simulink model "TRIAD"  (R2017a)
settings: Solver=ode4  StartTime=0.0  StopTime=20000  FixedStep=0.1  RelTol=1e-3  EnableMultiTasking=on
undefined symbols (not defined in the file): mbaseserialmask, RxBuffer
libraries: xpcseriallib x17, vrlib x7, slrtlib x4, sharedtransform x3, sharedutil x2, dspinverses x2, dspmathops x2, simulink x1, dspsigops x1
(part 3 of 3)

== matlab function TRIAD/TRIAD_inner_use_Projection/BODY_TRIAD ==
  data: v input; c_triad output; w input
function c_triad = fcn(v, w)
    nz = norm(v);
    if (nz == 0)
        c_triad = eye(3);
    else
        x = v/norm(v);
        z = cross(x, w);
        z = z/norm(z);
        y = cross(z, x);
        c_triad = [x'; y'; z'];
    end
end

== matlab function TRIAD/SUN_function/Subsystem8/MATLAB Function4 ==
  data: djm input; sunpos output; ts input
function sunpos  = sun (djm, ts)
% [sunpos] = sun (djm, ts)
%
%	The subroutine sun calculates the position vector
%	of the Sun in the geocentric inertial system refered
%	to j2000 equator and equinox.
%
% Input:
%	djm
%		modified julian date in days, referred to 1950.0.
%	ts
%		fraction of the day in seconds.
%
% Output:
%	sunpos
%		position vector of the sun:
%		(1) - first component of earth-sun position vector in meters.
%		(2) - second component of earth-sun position vector in meters.
%		(3) - third component of earth-sun position vector in meters.
%		(4) - right ascension in radians.
%		(5) - declination in radians.
%		(6) - radius vector (distance) in meters.
%
% Remarks:
%	this subroutine is optimized from 1950-1-1 00:01:06
%	until year 2050.
%
% Author:
%	Helio Koiti Kuga and Ulisses T. V. Guedes * version 1.0
%	C version by Valdemir Carrara 7/05
%   Valdemir Carrara            March/09        Matlab

rad = pi/180;
ASTRONOMICAL_UNIT	= 149.60e+09;		% Astronomical unit (meters)

t = djm - 18262.5 + ts/86400.;%86400:1day second 
                              %18262.5 : J2000년도 Jan1 day1  
%	Long. media do sol, corrigida

alom_ab = mod ((280.460 + 0.9856474*t)*rad, 2*pi);
% 280.460 = mean longitude of the sun
% alom_ab : meanlongitude
% Sun's mean anomaly
% site : https://forum.logicmachine.net/showthread.php?tid=510

% alom_ab = 280.461 + 0.9856474 * t;
% while (alom_ab<0)
%     alom_ab = alom_ab + 360.0;
% end

if alom_ab < 0
    alom_ab = alom_ab + 2*pi;
end
% http://webcache.googleusercontent.com/search?q=cache:http://www.astro.uni.torun.pl/~kb/AllSky-old/Docs/Top2B2.htm&gws_rd=cr&dcr=0&ei=MUuaWu_oHYyB8gXs_J-4Ag
%	Anomalia media
% https://en.wikipedia.org/wiki/Position_of_the_Sun
an_mean = mod ((357.528 + 0.9856003*t)*rad, 2*pi);
if an_mean < 0
    an_mean = an_mean + 2*pi;
end

an_mean_2 = an_mean +  an_mean;

if an_mean_2 > 2*pi
    an_mean_2 = mod (an_mean_2, 2*pi);
end

ecli_lo = alom_ab + (1.915*sin(an_mean) +0.02*sin(an_mean_2))*rad;
sin_ecli_lo = sin(ecli_lo);
cos_ecli_lo = cos(ecli_lo);

%	ecliptic latitude	ecli_la = 0

obl_ecli = (23.439 - 4.e-7*t)*rad; % tilt angle 23.439
sin_obl_ecli = sin(obl_ecli);
cos_obl_ecli = cos(obl_ecli);

sunpos = [0, 0, 0, 0, 0, 0];
sunpos(4)  = atan2(cos_obl_ecli*sin_ecli_lo, cos_ecli_lo);
if sunpos(4) < 0
    sunpos(4) = sunpos(4) + 2*pi;
end

sunpos(5) = asin(sin_obl_ecli*sin_ecli_lo);
sunpos(6) = (1.00014 - 0.01671*cos(an_mean) - 1.4e-4*cos(an_mean_2))*ASTRONOMICAL_UNIT;

sunpos(1) = sunpos(6) * cos_ecli_lo;
sunpos(2) = sunpos(6) * cos_obl_ecli * sin_ecli_lo;
sunpos(3) = sunpos(6) * sin_obl_ecli * sin_ecli_lo;
end

== matlab function TRIAD/SUN_function/Subsystem8/MATLAB Function5 ==
  data: u input; y output
function y = fcn(u)
y = u(1:3);

end

== matlab function TRIAD/SUN_function/Subsystem8/MATLAB Function2 ==
  data: sat_pos input; shadow output; sun_pos input
function shadow  = earth_shadow (sat_pos, sun_pos)
% [shadow] = earth_shadow (sat_pos, sun_pos)
%
%	The function earth_shadow verifies if a given position
%	is or isn't in the earth shadow.
%
% Inputs:
%	sat_pos
%		spacecraft coordinates in the inertial system, in meters.
%	sun_pos
%		coordinates of the sun in the inertial frame, in meters.
%
% Remarks:
%	1 - Earth is considered as a sphere
%	2 - Penunbra is calculated as straight horizon line
%
% Outputs:
%	earth_shadow
%		0: spacecraft is in the earth shadow
%		1: spacecraft is illuminated by the sun
%       between 0 and 1: spacecraft is in the Earth penumbra,
%		earth_shadow gives the visible fraction of the sun.
%
% Author:  Valdemir Carrara            mar/88        v. 1.0
%									july/05			C version
%   Valdemir Carrara            March/09        Matlab

EARTH_RADIUS	= 6378139.;		% Earth's radius in meters
SUN_RADIUS		= 0.6953e+09;	% Sun's radius (meters)

dsun   = norm(sun_pos(1:3));
if dsun <= 0
    shadow =  -1;	% a distancia ao Sol �nula
else
	vecsun = sun_pos(1:3)/dsun;
	rcob   = dot(sat_pos(1:3), vecsun);
	if rcob < 0
		radi   = SUN_RADIUS/dsun;
        auxi   = cross(sat_pos(1:3),vecsun);
        auxi   = norm(auxi);
		psvs   = (auxi - EARTH_RADIUS)/rcob/radi;
		if abs(psvs) < 1
            shadow = (acos(psvs) - psvs*sqrt(1. - psvs*psvs))/pi;
        else
            if psvs >= 0
                shadow = 0;
            else
                shadow = 1;
            end
        end
    else
        shadow = 1;
    end
end

== matlab function TRIAD/SUN_function/Subsystem8/MATLAB Function ==
  data: lat input; ecef_position output; lon input; alt input
function ecef_position = fcn(lat, lon, alt)

ecef_position = [(alt*cos(lat))*cos(lon), (alt*cos(lat))*sin(lon), alt*sin(lat)]';
end

== matlab function TRIAD/SUN_function/MATLAB Function ==
  data: measured_Sun_vector input; angle output; Body_z_axis input
function angle = fcn(measured_Sun_vector, Body_z_axis)
v_1 = measured_Sun_vector';
v_2 = Body_z_axis';
v_1 = v_1/norm(v_1);

angle = acos( dot(v_1,v_2)/(norm(v_1)*norm(v_2)) );

if angle > (40*(pi/180))
    angle = 41*(pi/180);
else
end
end

== matlab function TRIAD/SUN_function/MATLAB Function1 ==
  data: measured_Sun_vector input; angle output; Body_x_axis input
function angle = fcn(measured_Sun_vector, Body_x_axis)

temp_ = measured_Sun_vector';%othogonal_projection of measured_Sun_vector

v_1 = temp_(1:2);
v_2 = Body_x_axis(1:2);

v_1 = v_1/norm(v_1);

angle = (asin(v_1(1,1)*v_2(1,2) - v_2(1,1)*v_1(1,2)))/(norm(v_1)*norm(v_2));

end

== matlab function TRIAD/Subsystem/MATLAB Function ==
  data: sec input; hour output; min output; sec output
function [hour, min, sec] = fcn(sec)
    hour = floor(sec/3600);
    min  = floor((rem(sec,3600))/60);
    sec  = rem(sec,60);
end

== matlab function TRIAD/TRIAD_inner_use_Projection/Standard_TRIAD ==
  data: v input; c_triad output; w input
function c_triad = fcn(v, w)
    nz = norm(v);
    if (nz == 0)
        c_triad = eye(3);
    else
        x = v/norm(v);
        z = cross(x, w);
        z = z/norm(z);
        y = cross(z, x);
        c_triad = [x'; y'; z'];
    end
end

== matlab function TRIAD/TRIAD_inner_use_Projection/TIRAD_STA_BODY ==
  data: mat1 input; c_triad output; mat2 input
function c_triad = fcn(mat1, mat2)
c_triad = mat1'*mat2;
end

== matlab function TRIAD/Subsystem6/MATLAB Function4 ==
  data: Sat_position input; orbit_x output; orbit_y output; orbit_z output; saved input; Sat_position output
function [orbit_x, orbit_y, orbit_z, Sat_position]    = fcn(Sat_position,saved)
   orbit_x     = Sat_position - saved;
   orbit_z     = -1*Sat_position;
   orbit_y     = cross(orbit_z, orbit_x);
end

== matlab function TRIAD/Subsystem6/MATLAB Function5 ==
  data: lat input; ecef_position output; lon input; alt input
function ecef_position = fcn(lat, lon, alt)

ecef_position = [(alt*cos(lat))*cos(lon), (alt*cos(lat))*sin(lon), alt*sin(lat)]';
end

== matlab function TRIAD/Subsystem6/MATLAB Function6 ==
  data: orbit_x input; v_orbit output; orbit_y input; orbit_z input; ecef_v input
function v_orbit  = fcn(orbit_x,orbit_y,orbit_z,ecef_v)
v_orbit = zeros(1,3);

v_orbit(1,1) = dot(ecef_v' , (orbit_x / norm(orbit_x)));
v_orbit(1,2) = dot(ecef_v' , (orbit_y / norm(orbit_y)));
v_orbit(1,3) = dot(ecef_v' , (orbit_z / norm(orbit_z)));
end

== matlab function TRIAD/Subsystem1/MATLAB Function2 ==
  data: Sat_position input; orbit_x output; orbit_y output; orbit_z output; saved input; Sat_position output
function [orbit_x, orbit_y, orbit_z, Sat_position]    = fcn(Sat_position,saved)
   orbit_x     = Sat_position - saved;
   orbit_z     = -1*Sat_position;
   orbit_y     = cross(orbit_z, orbit_x);
end

== matlab function TRIAD/Subsystem1/MATLAB Function7 ==
  data: lat input; ecef_position output; lon input; alt input
function ecef_position = fcn(lat, lon, alt)

ecef_position = [(alt*cos(lat))*cos(lon), (alt*cos(lat))*sin(lon), alt*sin(lat)]';
end

== matlab function TRIAD/SUN_function/Subsystem8/Rotation matrix (ECI to ECEF) ==
  data: GMST input; mat output
function mat  = eci2ecef(GMST)

GMST  = rem(GMST,2*pi);

sGMST = sin(GMST);
cGMST = cos(GMST);

ROT_Z   = [      cGMST,  -1*sGMST, 0; 
                 sGMST,    cGMST , 0; 
                   0  ,      0   , 1];
mat =  ROT_Z;
              
end

== matlab function TRIAD/Subsystem6/MATLAB Function3 ==
  data: u input; y output
function y = fcn(u)
y = u(1:3);

end

== matlab function TRIAD/Subsystem1/Rotation matrix (ECEF to NED) ==
  data: mat output; lat input; lon input
function mat   = ECEF2NED(lat, lon)
% https://kr.mathworks.com/help/aeroblks/directioncosinematrixeceftoned.html
% [my_ned2ecef( n, e, d, lat, lon, alt )]
% lat, lon  : rad
    R1 = [-sin(lat), 0, cos(lat);
               0   , 1,    0    ;
          -cos(lat), 0,-sin(lat)
          ];
    R2 = [ cos(lon), sin(lon), 0;
          -sin(lon), cos(lon), 0;
               0   ,    0    , 1
         ];
    mat = R1 * R2; % This is DCM (From ECEF to NED)
    mat = mat';    % Convert to Rotation matrix
end

== matlab function TRIAD/SUN_function/Subsystem8/Subsystem7/Rotation matrix (ECI to ECEF) ==
  data: GMST input; mat output
function mat  = eci2ecef(GMST)

GMST  = rem(GMST,2*pi);

sGMST = sin(GMST);
cGMST = cos(GMST);

ROT_Z   = [      cGMST,  -1*sGMST, 0; 
                 sGMST,    cGMST , 0; 
                   0  ,      0   , 1];
mat =  ROT_Z;
              
end

== matlab function TRIAD/SUN_function/Subsystem8/Subsystem7/Rotation matrix (ECI to Perifocal) ==
  data: ke input; mat output
function mat = eci2perifocal( ke )
RAAN         = ke(4,1);%rem(ke(4,1),2*pi)
Arg_perigee  = ke(5,1);%rem(ke(5,1),2*pi)
inclination  = ke(3,1);%rem(ke(3,1),2*pi);

% theta1 = (RAAN + Arg_perigee);%rem((RAAN + Arg_perigee),2*pi);
R1 = [   cos(RAAN),  -sin(RAAN), 0;
         sin(RAAN),   cos(RAAN), 0;
             0    ,       0    , 1 ];
             
R2 = [      1,          0    ,           0;
            0,     cos(inclination),    -sin(inclination);
            0,     sin(inclination),       cos(inclination)];
        
R3 = [   cos(Arg_perigee),  -sin(Arg_perigee), 0;
         sin(Arg_perigee),   cos(Arg_perigee), 0;
                0        ,           0       , 1];
             
mat = R1 * R2 * R3;
end

== matlab function TRIAD/SUN_function/Subsystem8/Subsystem7/Rotation matrix (Perifocal to Orbit) ==
  data: ke input; mat output
function mat = perifocal2orbit( ke )
% 		vector with the keplerian elements:
%		(1) - semimajor axis of the orbit in meters.
%		(2) - eccentricity.
%		(3) - inclination in radians.
%		(4) - right ascension of ascending node in radians.
%		(5) - argument of perigee in radians.
%		(6) - mean anomaly in radians.
mean_anomaly = ke(6,1);
%theta = rem(mean_anomaly,2*pi);

R1 = [ cos(mean_anomaly + pi/2),-sin(mean_anomaly + pi/2), 0;
       sin(mean_anomaly + pi/2), cos(mean_anomaly + pi/2), 0;
             0        ,         0        , 1    ];
R2 = [  1,     0     ,      0     ; 
        0, cos(-pi/2), -sin(-pi/2);
        0, sin(-pi/2),  cos(-pi/2)];

mat = R1 * R2;

end
